simulink model "robot_4DOF_jointspace_controllerdesign"  (Simulink 7.3)
settings: Solver=ode4  StartTime=0.0  StopTime=.5  FixedStep=.002  MinStep=.002  RelTol=1e-3
values from neighbouring files (symbols this model uses):
  Kp = [60;50;40;40]*25    [Control1.m]    (also in dynamics_4DOF.m = [60;40;20;10]; dynamics_4DOF_loop_taskoriented.m = 5*[60;50;40;40])
  Kv = 8*[8 8 7 7]'    [Control1.m]    (also in dynamics_4DOF.m = [5 6 7 5]'; dynamics_4DOF_loop_taskoriented.m = 12*[10 7 7 6]')
libraries: simulink_extras x1, sdolib x1, dspinverses x1
settings Model: Creator=arash  LastModifiedBy=arash
settings SolverCC: ExtrapolationOrder=1

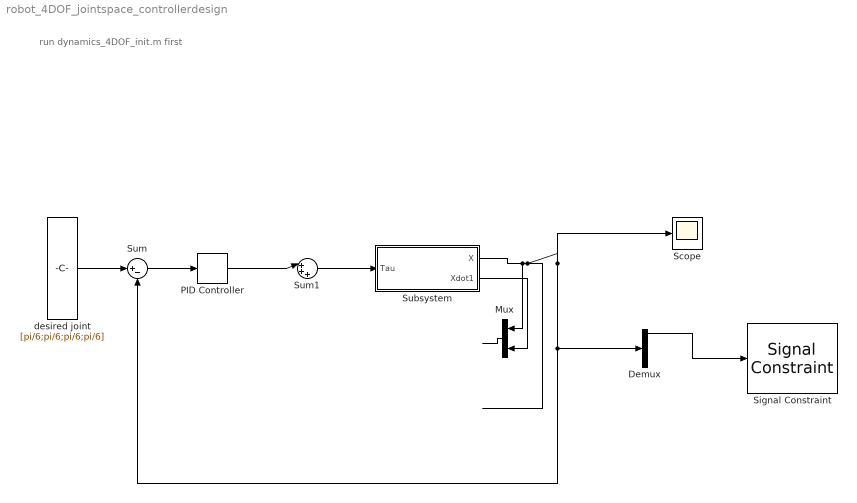
== system robot_4DOF_jointspace_controllerdesign ==
  note: run dynamics_4DOF_init.m first
  Demux : Demux
  Mux : Mux  Inputs=2
  PID Controller : simulink_extras/Additional Linear/PID Controller  SystemSampleTime=-1  P=Kp  I=[0;0;0;0]  D=Kv
  Scope : Scope
      settings: YMin=-1  YMax=1
  Signal Constraint : sdolib/Signal Constraint  SystemSampleTime=-1  DialogPosition=[0.46015625 0.0825 0.45 0.31]  SaveIn=workspace  SaveAs=robot_4DOF_jointspace_controllerdesign_optim  LogID=SRO_DataLog_1
  Subsystem : Subsystem
  Sum : Sum  Inputs=|+-  OutDataType=fixdt(1, 16)  OutScaling=2^0
  Sum1 : Sum  Inputs=|+++  OutDataType=fixdt(1, 16)  OutScaling=2^0
  desired joint : Constant  Value=[pi/6;pi/6;pi/6;pi/6]  OutDataType=fixdt(1, 16)  OutScaling=2^0
  wires:
  desired joint/1 -> Sum/1
  Subsystem/1(X) -> Scope/1, Sum/2, Demux/1, Mux/1
  Sum/1 -> PID Controller/1
  Sum1/1 -> Subsystem/1(Tau)
  PID Controller/1 -> Sum1/1
  ? -> Sum1/2
  ? -> Sum1/3
  Mux/1 -> ?
  Subsystem/2(Xdot1) -> Mux/2
  Demux/1 -> Signal Constraint/1

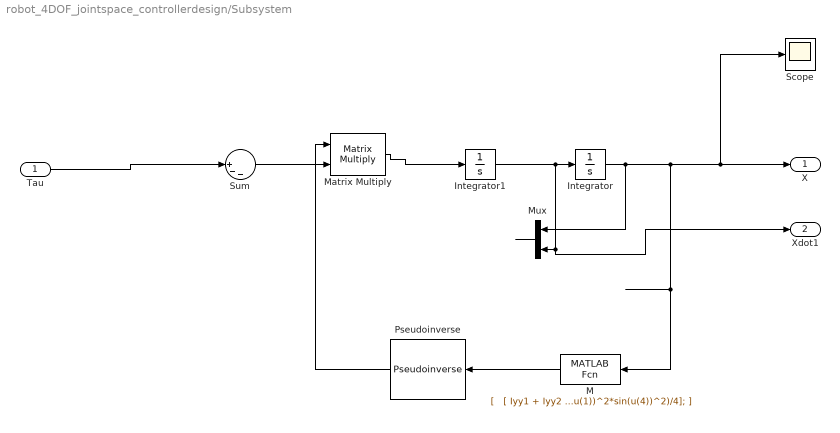
== system robot_4DOF_jointspace_controllerdesign/Subsystem ==
  Tau : Inport  OutDataType=fixdt(1, 16)  OutScaling=2^0
  Integrator : Integrator  ZeroCross=off
  Integrator1 : Integrator  ZeroCross=off
  M : MATLABFcn  MATLABFcn=|  OutputDimensions=[4 4]  OutputSignalType=real  Output1D=off
      | [
      |  
      | [ Iyy1 + Iyy2 + 1.0*Iyy3 + (m3*(2*(1.0*l2*sin(u(1) + u(2)) + l1*sin(u(1)) + 0.5*l3*sin(u(1) + u(2) + u(3)))*(l2*sin(u(1) + u(2)) + l1*sin(u(1)) + (l3*sin(u(1) + u(2) + u(3)))/2)*cos(u(4))^2 + 2*(1.0*l2*sin(u(1) + u(2)) + l1*sin(u(1)) + 0.5*l3*sin(u(1) + u(2) + u(3)))*(l2*sin(u(1) + u(2)) + l1*sin(u(1)) + (l3*sin(u(1) + u(2) + u(3)))/2)*sin(u(4))^2 + 2*(l2*cos(u(1) + u(2)) + l1*cos(u(1)) + (l3*cos(u(1) + u(2) + u(3)))/2)*(1.0*l2*cos(u(1) + u(2)) + l1*cos(u(1)) + 0.5*l3*cos(u(1) + u(2) + u(3)))))/2 + (l1^2*m1)/4 + (m2*(2*((l2*sin(u(1) + u(2)))/2 + l1*sin(u(1)))*(0.5*l2*sin(u(1) + u(2)) + l1*sin(u(1)))*cos(u(4))^2 + 2*((l2*sin(u(1) + u(2)))/2 + l1*sin(u(1)))*(0.5*l2*sin(u(1) + u(2)) + l1*sin(u(1)))*sin(u(4))^2 + 2*((l2*cos(u(1) + u(2)))/2 + l1*cos(u(1)))*(0.5*l2*cos(u(1) + u(2)) + l1*cos(u(1)))))/2, Iyy2 + 1.0*Iyy3 + (m3*(2*(1.0*l2*sin(u(1) + u(2)) + 0.5*l3*sin(u(1) + u(2) + u(3)))*(l2*sin(u(1) + u(2)) + l1*sin(u(1)) + (l3*sin(u(1) + u(2) + u(3)))/2)*cos(u(4))^2 + 2*(1.0*l2*sin(u(1) + u(2)) + 0.5*l3*sin(u(1) + u(2) + u(3)))*(l2*sin(u(1) + u(2)) + l1*sin(u(1)) + (l3*sin(u(1) + u(2) + u(3)))/2)*sin(u(4))^2 + 2*(1.0*l2*cos(u(1) + u(2)) + 0.5*l3*cos(u(1) + u(2) + u(3)))*(l2*cos(u(1) + u(2)) + l1*cos(u(1)) + (l3*cos(u(1) + u(2) + u(3)))/2)))/2 + (m2*(1.0*l2*sin(u(1) + u(2))*((l2*sin(u(1) + u(2)))/2 + l1*sin(u(1)))*cos(u(4))^2 + 1.0*l2*sin(u(1) + u(2))*((l2*sin(u(1) + u(2)))/2 + l1*sin(u(1)))*sin(u(4))^2 + 1.0*l2*cos(u(1) + u(2))*((l2*cos(u(1) + u(2)))/2 + l1*cos(u(1)))))/2, 1.0*Iyy3 + (m3*(1.0*l3*sin(u(1) + u(2) + u(3))*(l2*sin(u(1) + u(2)) + l1*sin(u(1)) + (l3*sin(u(1) + u(2) + u(3)))/2)*cos(u(4))^2 + 1.0*l3*sin(u(1) + u(2) + u(3))*(l2*sin(u(1) + u(2)) + l1*sin(u(1)) + (l3*sin(u(1) + u(2) + u(3)))/2)*sin(u(4))^2 + 1.0*l3*cos(u(1) + u(2) + u(3))*(l2*cos(u(1) + u(2)) + l1*cos(u(1)) + (l3*cos(u(1) + u(2) + u(3)))/2)))/2,                                                                                                                                                                                                                                                                                                                                                                                                                                                                                                                                                                                    0];
      | [                                                                                                                                                                                                                                                                                                                                                                                                                                                                                                                                                                                                                                                                                 Iyy2 + Iyy3 + (l2^2*m2)/4 + l2^2*m3 + (l3^2*m3)/4 + (l1*l3*m3*cos(u(2) + u(3)))/2 + (l1*l2*m2*cos(u(2)))/2 + l1*l2*m3*cos(u(2)) + l2*l3*m3*cos(u(3)),                                                                                                                                                                                                                                                                                                                                                                                                                                                                                                                                                                                                                                    Iyy2 + Iyy3 + (l2^2*m2)/4 + l2^2*m3 + (l3^2*m3)/4 + l2*l3*m3*cos(u(3)),                                                                                                                                                                                                                                                                                                                    (m3*l3^2)/4 + (l2*m3*cos(u(3))*l3)/2 + Iyy3,                                                                                                                                                                                                                                                                                                                                                                                                                                                                                                                                                                                    0];
      | [                                                                                                                                                                                                                                                                                                                                                                                                                                                                                                                                                                                                                                                                                                                                                          Iyy3 + (l3^2*m3)/4 + (l1*l3*m3*cos(u(2) + u(3)))/2 + (l2*l3*m3*cos(u(3)))/2,                                                                                                                                                                                                                                                                                                                                                                                                                                                                                                                                                                                                                                                               (m3*l3^2)/4 + (l2*m3*cos(u(3))*l3)/2 + Iyy3,                                                                                                                                                                                                                                                                                                                                             (m3*l3^2)/4 + Iyy3,                                                                                                                                                                                                                                                                                                                                                                                                                                                                                                                                                                                    0];
      | [                                                                                                                                                                                                                                                                                                                                                                                                                                                                                                                                                                                                                                                                                                                                                                                                                                    0,                                                                                                                                                                                                                                                                                                                                                                                                                                                                                                                                                                                                                                                                                                         0,                                                                                                                                                                                                                                                                                                                                                              0, I4 - Izz2*(cos(u(1) + u(2))^2 - 1) + (m2*(2*cos(u(4))^2*((l2*cos(u(1) + u(2)))/2 + l1*cos(u(1)))^2 + 2*sin(u(4))^2*((l2*cos(u(1) + u(2)))/2 + l1*cos(u(1)))^2))/2 + Ixx3*cos(u(1) + u(2) + u(3))^2 - Izz1*(cos(u(1))^2 - 1) - Izz3*(cos(u(1) + u(2) + u(3))^2 - 1) + Ixx2*cos(u(1) + u(2))^2 + Ixx1*cos(u(1))^2 + (m3*(2*cos(u(4))^2*(l2*cos(u(1) + u(2)) + l1*cos(u(1)) + (l3*cos(u(1) + u(2) + u(3)))/2)^2 + 2*sin(u(4))^2*(l2*cos(u(1) + u(2)) + l1*cos(u(1)) + (l3*cos(u(1) + u(2) + u(3)))/2)^2))/2 + (l1^2*m1*cos(u(1))^2*cos(u(4))^2)/4 + (l1^2*m1*cos(u(1))^2*sin(u(4))^2)/4];
      | ]
  Matrix Multiply : Product  Multiplication=Matrix(*)  OutDataType=sfix(16)  OutScaling=2^0
  Mux : Mux  Inputs=2
  Pseudoinverse : dspinverses/Pseudoinverse  wanterr=off
  Scope : Scope
      settings: YMin=-2.75  YMax=0.25
  Sum : Sum  Inputs=||+--  OutDataType=fixdt(1, 16)  OutScaling=2^0
  X : Outport  OutDataType=fixdt(1, 16)  OutScaling=2^0
  Xdot1 : Outport  Port=2  OutDataType=fixdt(1, 16)  OutScaling=2^0
  wires:
  Integrator/1 -> Mux/1, M/1, X/1, Scope/1
  Integrator1/1 -> Mux/2, Xdot1/1, Integrator/1
  Mux/1 -> ?
  M/1 -> Pseudoinverse/1
  ? -> Sum/3
  ? -> Sum/2
  Sum/1 -> Matrix Multiply/2
  Matrix Multiply/1 -> Integrator1/1
  Pseudoinverse/1 -> Matrix Multiply/1
  Tau/1 -> Sum/1
